simulink model "actividad5"  (Simulink 7.9)
settings: Solver=ode45  StartTime=0.0  StopTime=10.0  RelTol=1e-3
settings Model: Creator=root  LastModifiedBy=root

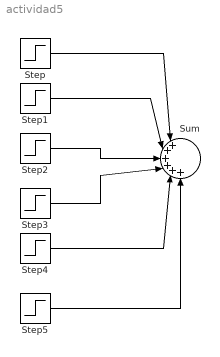
== system actividad5 ==
  Step{,1..5} (6 alike) : Step  SampleTime=0
  Sum : Sum  Inputs=|++++++
  wires:
  Step/1 -> Sum/1
  Step1/1 -> Sum/2
  Step2/1 -> Sum/3
  Step3/1 -> Sum/4
  Step4/1 -> Sum/5
  Step5/1 -> Sum/6
